simulink library "contactlib"  (R2013b)
settings: Solver=ode45  StartTime=0.0  StopTime=10.0  RelTol=1e-3
undefined symbols (not defined in the file): rWheel
libraries: nesl_utility x29, sm_lib x17, contactlib x4, dspinverses x2, contact3D_lib x2
settings Model: Creator=scastro  LastModifiedBy=scastro

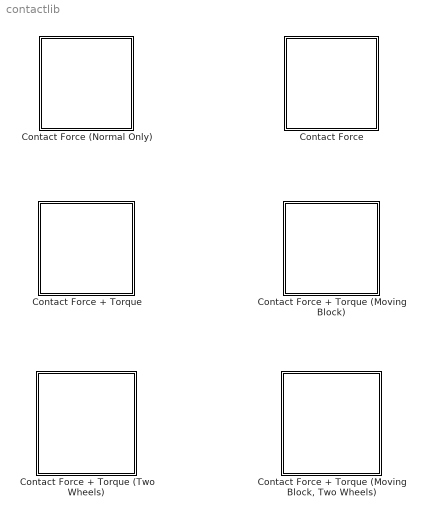
== system contactlib ==
  Contact Force : Subsystem  mask{rWheel=1, k=300000, b=5000, xBlock=2, yBlock=5, zBlock=0.2}
      mask prompts: rWheel "Wheel Radius [m]"; k "Contact Stiffness"; b "Contact Damping"; xBlock "Block X [m]"; yBlock "Block Y [m]"; zBlock "Block Z [m]"
  Contact Force (Normal Only) : Subsystem  mask{rWheel=1, k=500000, b=20000, xBlock=2, yBlock=3, zBlock=0.2}
      mask prompts: rWheel "Wheel Radius [m]"; k "Contact Stiffness"; b "Contact Damping"; xBlock "Block X [m]"; yBlock "Block Y [m]"; zBlock "Block Z [m]"
  Contact Force + Torque : Subsystem  mask{rWheel=rWheel, k=2500, b=100, b2=1000, xBlock=2, yBlock=3.5, zBlock=0.2}
      mask prompts: rWheel "Wheel Radius [m]"; k "Contact Stiffness"; b "Contact Damping"; b2 "Slip Damping"; xBlock "Block X [m]"; yBlock "Block Y [m]"; zBlock "Block Z [m]"
  Contact Force + Torque (Moving Block) : Subsystem  mask{rWheel=rWheel, k=2500, b=100, b2=0, xBlock=2, yBlock=3.5, zBlock=0.2}
      mask prompts: rWheel "Wheel Radius [m]"; k "Contact Stiffness"; b "Contact Damping"; b2 "Slip Damping"; xBlock "Block X [m]"; yBlock "Block Y [m]"; zBlock "Block Z [m]"
  "Contact Force + Torque (Moving Block, Two Wheels)" : Subsystem  AncestorBlock=|  mask{rWheel=0, k=0, b=0, b2=0, xBlock=0, yBlock=0, zBlock=0}
      | contactlib/Contact Force + Torque
      | (Two Wheels)
      mask prompts: rWheel "Wheel Radius [m]"; k "Contact Stiffness"; b "Contact Damping"; b2 "Slip Damping"; xBlock "Block X [m]"; yBlock "Block Y [m]"; zBlock "Block Z [m]"
  Contact Force + Torque (Two Wheels) : Subsystem  mask{rWheel=0, k=0, b=0, b2=0, xBlock=0, yBlock=0, zBlock=0}
      mask prompts: rWheel "Wheel Radius [m]"; k "Contact Stiffness"; b "Contact Damping"; b2 "Slip Damping"; xBlock "Block X [m]"; yBlock "Block Y [m]"; zBlock "Block Z [m]"

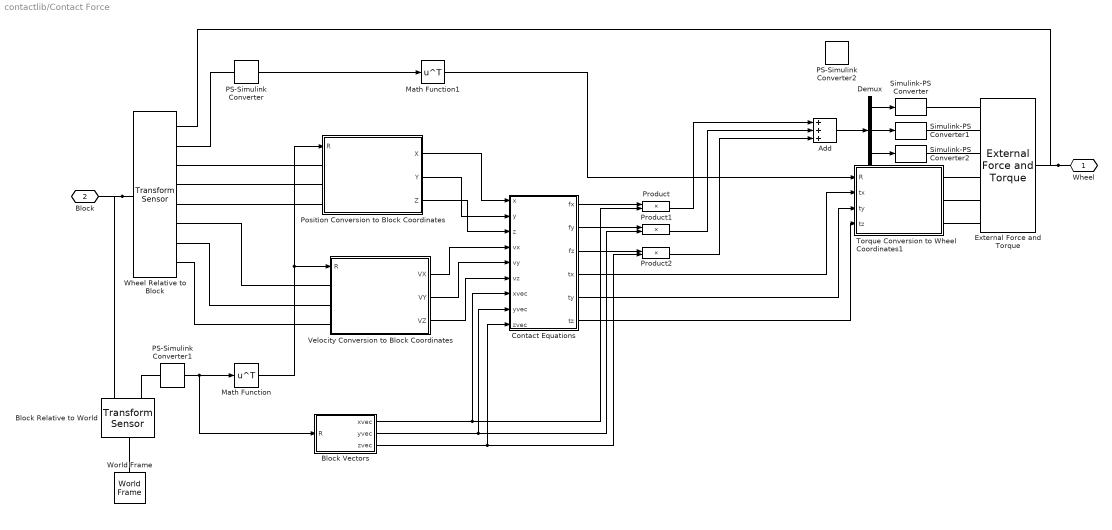
== system contactlib/Contact Force ==
  Add : Sum  Inputs=+++
  Block Relative to World : sm_lib/Frames and Transforms/Transform Sensor  MeasurementFrame=Base  SenseAngle=off  SenseAxis=off  SenseAngle1=off  SenseAngle2=off  SenseAngle3=off  SenseQ=off  SenseR=on  SenseOmegaX=off  SenseOmegaY=off  SenseOmegaZ=off  SenseOmega1=off  SenseOmega2=off  SenseOmega3=off  SenseQDot=off  SenseRDot=off  SenseAlphaX=off  SenseAlphaY=off  SenseAlphaZ=off  SenseAlpha1=off  SenseAlpha2=off  SenseAlpha3=off  SenseQDDot=off  SenseRDDot=off  SenseX=off  SenseY=off  SenseZ=off  SenseRad=off  SenseAzim=off  SenseDist=off  SenseInc=off  SenseXDot=off  SenseYDot=off  SenseZDot=off  SenseRadDot=off  SenseAzimDot=off  SenseDistDot=off  SenseIncDot=off  SenseXDDot=off  SenseYDDot=off  SenseZDDot=off  SenseRadDDot=off  SenseAzimDDot=off  SenseDistDDot=off  SenseIncDDot=off  BlockFunction=simmechanics.library.frames_transforms.transform_sensor
  Block Vectors : Subsystem
  Contact Equations : MATLAB Function  TreatAsAtomicUnit=on
  Demux : Demux  Outputs=3
  External Force and Torque : sm_lib/Forces and Torques/External Force and Torque  ForceResolutionFrame=World  EnableForceX=on  EnableForceY=on  EnableForceZ=on  EnableForce=off  TorqueResolutionFrame=AttachedFrame  EnableTorqueX=on  EnableTorqueY=on  EnableTorqueZ=on  EnableTorque=off  BlockFunction=simmechanics.library.forces_torques.external_force_torque
  Math Function : Math  Operator=transpose  SaturateOnIntegerOverflow=on
  Math Function1 : Math  Operator=transpose  SaturateOnIntegerOverflow=on
  PS-Simulink Converter : nesl_utility/PS-Simulink Converter  PhysicalDomain=network_engine_domain  SubClassName=ps_output  LeftPortType=input  RightPortType=output  PseudoPeriodic=off  Frequencies=[]  Unit=1  AffineConversion=off
  PS-Simulink Converter1 : nesl_utility/PS-Simulink Converter  PhysicalDomain=network_engine_domain  SubClassName=ps_output  LeftPortType=input  RightPortType=output  PseudoPeriodic=off  Frequencies=[]  Unit=1  AffineConversion=off
  PS-Simulink Converter2 : nesl_utility/PS-Simulink Converter  PhysicalDomain=network_engine_domain  SubClassName=ps_output  LeftPortType=input  RightPortType=output  PseudoPeriodic=off  Frequencies=[]  Unit=1  AffineConversion=off
  Position Conversion to Block Coordinates : Subsystem
  Product : Product
  Product1 : Product
  Product2 : Product
  Simulink-PS Converter : nesl_utility/Simulink-PS Converter  PhysicalDomain=network_engine_domain  SubClassName=ps_input  LeftPortType=input  RightPortType=output  PseudoPeriodic=off  Frequencies=[]  NoiseDistribution=none  NoiseParameters=[]  Unit=1  AffineConversion=off  InputFiltering=off  SimscapeFilterOrder=1  InputFilterTimeConstant=0.001  UdotUserProvided=1
  Simulink-PS Converter1 : nesl_utility/Simulink-PS Converter  PhysicalDomain=network_engine_domain  SubClassName=ps_input  LeftPortType=input  RightPortType=output  PseudoPeriodic=off  Frequencies=[]  NoiseDistribution=none  NoiseParameters=[]  Unit=1  AffineConversion=off  InputFiltering=off  SimscapeFilterOrder=1  InputFilterTimeConstant=0.001  UdotUserProvided=1
  Simulink-PS Converter2 : nesl_utility/Simulink-PS Converter  PhysicalDomain=network_engine_domain  SubClassName=ps_input  LeftPortType=input  RightPortType=output  PseudoPeriodic=off  Frequencies=[]  NoiseDistribution=none  NoiseParameters=[]  Unit=1  AffineConversion=off  InputFiltering=off  SimscapeFilterOrder=1  InputFilterTimeConstant=0.001  UdotUserProvided=1
  Torque Conversion to Wheel Coordinates1 : Subsystem
  Velocity Conversion to Block Coordinates : Subsystem
  Wheel Relative to Block : sm_lib/Frames and Transforms/Transform Sensor  MeasurementFrame=World  SenseAngle=off  SenseAxis=off  SenseAngle1=off  SenseAngle2=off  SenseAngle3=off  SenseQ=off  SenseR=on  SenseOmegaX=off  SenseOmegaY=off  SenseOmegaZ=off  SenseOmega1=off  SenseOmega2=off  SenseOmega3=off  SenseQDot=off  SenseRDot=off  SenseAlphaX=off  SenseAlphaY=off  SenseAlphaZ=off  SenseAlpha1=off  SenseAlpha2=off  SenseAlpha3=off  SenseQDDot=off  SenseRDDot=off  SenseX=on  SenseY=on  SenseZ=on  SenseRad=off  SenseAzim=off  SenseDist=off  SenseInc=off  SenseXDot=on  SenseYDot=on  SenseZDot=on  SenseRadDot=off  SenseAzimDot=off  SenseDistDot=off  SenseIncDot=off  SenseXDDot=off  SenseYDDot=off  SenseZDDot=off  SenseRadDDot=off  SenseAzimDDot=off  SenseDistDDot=off  SenseIncDDot=off  BlockFunction=simmechanics.library.frames_transforms.transform_sensor
  World Frame : sm_lib/Frames and Transforms/World Frame  BlockFunction=simmechanics.library.frames_transforms.world_frame
  Wheel : PMIOPort  Port=1  Side=Right
  Block : PMIOPort  Port=2  Side=Left
  wires:
  Math Function/1 -> Velocity Conversion to Block Coordinates/1(R), Position Conversion to Block Coordinates/1(R)
  PS-Simulink Converter1/1 -> Math Function/1, Block Vectors/1(R)
  Math Function1/1 -> Torque Conversion to Wheel Coordinates1/1(R)
  PS-Simulink Converter/1 -> Math Function1/1
  Contact Equations/3(fz) -> Product2/1
  Contact Equations/2(fy) -> Product1/1
  Contact Equations/1(fx) -> Product/1
  Velocity Conversion to Block Coordinates/3(VZ) -> Contact Equations/6(vz)
  Velocity Conversion to Block Coordinates/2(VY) -> Contact Equations/5(vy)
  Velocity Conversion to Block Coordinates/1(VX) -> Contact Equations/4(vx)
  Position Conversion to Block Coordinates/3(Z) -> Contact Equations/3(z)
  Position Conversion to Block Coordinates/2(Y) -> Contact Equations/2(y)
  Position Conversion to Block Coordinates/1(X) -> Contact Equations/1(x)
  Block Vectors/1(xvec) -> Contact Equations/7(xvec), Product/2
  Block Vectors/2(yvec) -> Contact Equations/8(yvec), Product1/2
  Block Vectors/3(zvec) -> Contact Equations/9(zvec), Product2/2
  Product/1 -> Add/1
  Product1/1 -> Add/2
  Product2/1 -> Add/3
  Add/1 -> Demux/1
  Demux/1 -> Simulink-PS Converter/1
  Demux/2 -> Simulink-PS Converter1/1
  Demux/3 -> Simulink-PS Converter2/1
  Contact Equations/4(tx) -> Torque Conversion to Wheel Coordinates1/2(tx)
  Contact Equations/5(ty) -> Torque Conversion to Wheel Coordinates1/3(ty)
  Contact Equations/6(tz) -> Torque Conversion to Wheel Coordinates1/4(tz)
  connections:
  Block Relative to World/RConn2 -- PS-Simulink Converter1/LConn1
  Wheel Relative to Block/RConn8 -- Velocity Conversion to Block Coordinates/LConn3
  Velocity Conversion to Block Coordinates/LConn2 -- Wheel Relative to Block/RConn7
  Wheel Relative to Block/RConn6 -- Velocity Conversion to Block Coordinates/LConn1
  Wheel Relative to Block/RConn5 -- Position Conversion to Block Coordinates/LConn3
  Position Conversion to Block Coordinates/LConn2 -- Wheel Relative to Block/RConn4
  Position Conversion to Block Coordinates/LConn1 -- Wheel Relative to Block/RConn3
  Wheel Relative to Block/RConn2 -- PS-Simulink Converter/LConn1
  Wheel Relative to Block/LConn1 -- Block Relative to World/RConn1 -- Block/RConn1
  Wheel/RConn1 -- Wheel Relative to Block/RConn1 -- External Force and Torque/RConn1
  Simulink-PS Converter/RConn1 -- External Force and Torque/LConn1
  Simulink-PS Converter1/RConn1 -- External Force and Torque/LConn2
  Simulink-PS Converter2/RConn1 -- External Force and Torque/LConn3
  Torque Conversion to Wheel Coordinates1/RConn1 -- External Force and Torque/LConn4
  External Force and Torque/LConn5 -- Torque Conversion to Wheel Coordinates1/RConn2
  Torque Conversion to Wheel Coordinates1/RConn3 -- External Force and Torque/LConn6
  World Frame/RConn1 -- Block Relative to World/LConn1

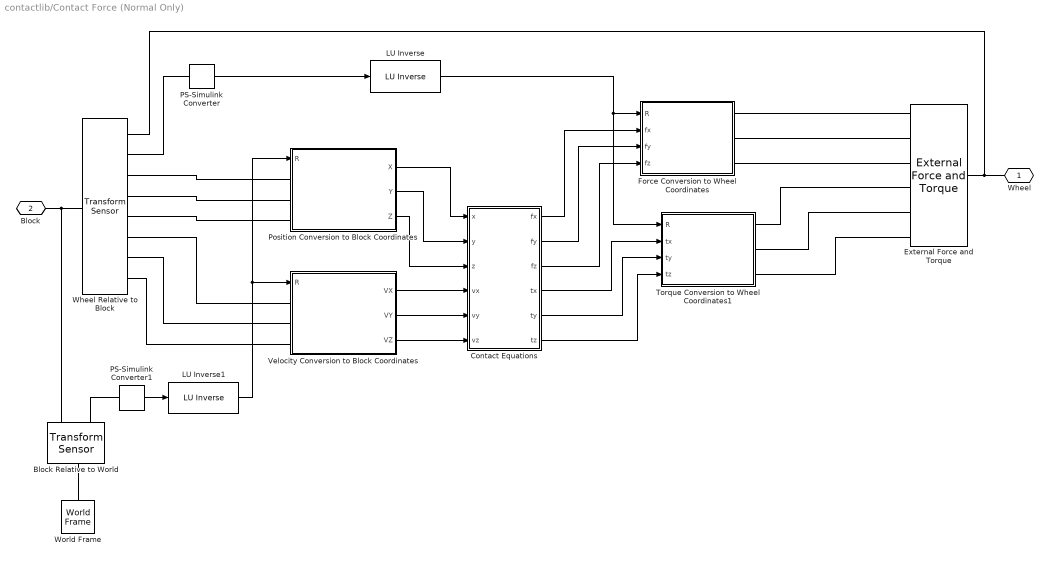
== system contactlib/Contact Force (Normal Only) ==
  " LU Inverse" : dspinverses/ LU Inverse
  " LU Inverse1" : dspinverses/ LU Inverse
  Block Relative to World : sm_lib/Frames and Transforms/Transform Sensor  MeasurementFrame=Base  SenseAngle=off  SenseAxis=off  SenseAngle1=off  SenseAngle2=off  SenseAngle3=off  SenseQ=off  SenseR=on  SenseOmegaX=off  SenseOmegaY=off  SenseOmegaZ=off  SenseOmega1=off  SenseOmega2=off  SenseOmega3=off  SenseQDot=off  SenseRDot=off  SenseAlphaX=off  SenseAlphaY=off  SenseAlphaZ=off  SenseAlpha1=off  SenseAlpha2=off  SenseAlpha3=off  SenseQDDot=off  SenseRDDot=off  SenseX=off  SenseY=off  SenseZ=off  SenseRad=off  SenseAzim=off  SenseDist=off  SenseInc=off  SenseXDot=off  SenseYDot=off  SenseZDot=off  SenseRadDot=off  SenseAzimDot=off  SenseDistDot=off  SenseIncDot=off  SenseXDDot=off  SenseYDDot=off  SenseZDDot=off  SenseRadDDot=off  SenseAzimDDot=off  SenseDistDDot=off  SenseIncDDot=off  BlockFunction=simmechanics.library.frames_transforms.transform_sensor
  Contact Equations : MATLAB Function  TreatAsAtomicUnit=on
  External Force and Torque : sm_lib/Forces and Torques/External Force and Torque  ForceResolutionFrame=AttachedFrame  EnableForceX=on  EnableForceY=on  EnableForceZ=on  EnableForce=off  TorqueResolutionFrame=AttachedFrame  EnableTorqueX=on  EnableTorqueY=on  EnableTorqueZ=on  EnableTorque=off  BlockFunction=simmechanics.library.forces_torques.external_force_torque
  Force Conversion to Wheel Coordinates : Subsystem
  PS-Simulink Converter : nesl_utility/PS-Simulink Converter  PhysicalDomain=network_engine_domain  SubClassName=ps_output  LeftPortType=input  RightPortType=output  PseudoPeriodic=off  Frequencies=[]  Unit=1  AffineConversion=off
  PS-Simulink Converter1 : nesl_utility/PS-Simulink Converter  PhysicalDomain=network_engine_domain  SubClassName=ps_output  LeftPortType=input  RightPortType=output  PseudoPeriodic=off  Frequencies=[]  Unit=1  AffineConversion=off
  Position Conversion to Block Coordinates : Subsystem
  Torque Conversion to Wheel Coordinates1 : Subsystem
  Velocity Conversion to Block Coordinates : Subsystem
  Wheel Relative to Block : sm_lib/Frames and Transforms/Transform Sensor  MeasurementFrame=World  SenseAngle=off  SenseAxis=off  SenseAngle1=off  SenseAngle2=off  SenseAngle3=off  SenseQ=off  SenseR=on  SenseOmegaX=off  SenseOmegaY=off  SenseOmegaZ=off  SenseOmega1=off  SenseOmega2=off  SenseOmega3=off  SenseQDot=off  SenseRDot=off  SenseAlphaX=off  SenseAlphaY=off  SenseAlphaZ=off  SenseAlpha1=off  SenseAlpha2=off  SenseAlpha3=off  SenseQDDot=off  SenseRDDot=off  SenseX=on  SenseY=on  SenseZ=on  SenseRad=off  SenseAzim=off  SenseDist=off  SenseInc=off  SenseXDot=on  SenseYDot=on  SenseZDot=on  SenseRadDot=off  SenseAzimDot=off  SenseDistDot=off  SenseIncDot=off  SenseXDDot=off  SenseYDDot=off  SenseZDDot=off  SenseRadDDot=off  SenseAzimDDot=off  SenseDistDDot=off  SenseIncDDot=off  BlockFunction=simmechanics.library.frames_transforms.transform_sensor
  World Frame : sm_lib/Frames and Transforms/World Frame  BlockFunction=simmechanics.library.frames_transforms.world_frame
  Wheel : PMIOPort  Port=1  Side=Right
  Block : PMIOPort  Port=2  Side=Left
  wires:
  Position Conversion to Block Coordinates/1(X) -> Contact Equations/1(x)
  Position Conversion to Block Coordinates/2(Y) -> Contact Equations/2(y)
  Position Conversion to Block Coordinates/3(Z) -> Contact Equations/3(z)
  Velocity Conversion to Block Coordinates/1(VX) -> Contact Equations/4(vx)
  Velocity Conversion to Block Coordinates/2(VY) -> Contact Equations/5(vy)
  Velocity Conversion to Block Coordinates/3(VZ) -> Contact Equations/6(vz)
  Contact Equations/1(fx) -> Force Conversion to Wheel Coordinates/2(fx)
  Contact Equations/2(fy) -> Force Conversion to Wheel Coordinates/3(fy)
  Contact Equations/3(fz) -> Force Conversion to Wheel Coordinates/4(fz)
  PS-Simulink Converter/1 -> " LU Inverse"/1
  " LU Inverse"/1 -> Torque Conversion to Wheel Coordinates1/1(R), Force Conversion to Wheel Coordinates/1(R)
  PS-Simulink Converter1/1 -> " LU Inverse1"/1
  Contact Equations/4(tx) -> Torque Conversion to Wheel Coordinates1/2(tx)
  Contact Equations/5(ty) -> Torque Conversion to Wheel Coordinates1/3(ty)
  Contact Equations/6(tz) -> Torque Conversion to Wheel Coordinates1/4(tz)
  " LU Inverse1"/1 -> Position Conversion to Block Coordinates/1(R), Velocity Conversion to Block Coordinates/1(R)
  connections:
  External Force and Torque/RConn1 -- Wheel Relative to Block/RConn1 -- Wheel/RConn1
  Block/RConn1 -- Block Relative to World/RConn1 -- Wheel Relative to Block/LConn1
  Wheel Relative to Block/RConn2 -- PS-Simulink Converter/LConn1
  Position Conversion to Block Coordinates/LConn1 -- Wheel Relative to Block/RConn3
  Position Conversion to Block Coordinates/LConn2 -- Wheel Relative to Block/RConn4
  Wheel Relative to Block/RConn5 -- Position Conversion to Block Coordinates/LConn3
  Wheel Relative to Block/RConn6 -- Velocity Conversion to Block Coordinates/LConn1
  Velocity Conversion to Block Coordinates/LConn2 -- Wheel Relative to Block/RConn7
  Wheel Relative to Block/RConn8 -- Velocity Conversion to Block Coordinates/LConn3
  Force Conversion to Wheel Coordinates/RConn1 -- External Force and Torque/LConn1
  Force Conversion to Wheel Coordinates/RConn2 -- External Force and Torque/LConn2
  External Force and Torque/LConn3 -- Force Conversion to Wheel Coordinates/RConn3
  World Frame/RConn1 -- Block Relative to World/LConn1
  Block Relative to World/RConn2 -- PS-Simulink Converter1/LConn1
  Torque Conversion to Wheel Coordinates1/RConn3 -- External Force and Torque/LConn6
  Torque Conversion to Wheel Coordinates1/RConn1 -- External Force and Torque/LConn4
  External Force and Torque/LConn5 -- Torque Conversion to Wheel Coordinates1/RConn2

== system contactlib/Contact Force + Torque ==
  Ball To Box 3D Contact : contact3D_lib/Ball To Box 3D Contact  rWheel=rWheel m  xBlock=xBlock m  yBlock=yBlock m  zBlock=zBlock m  k=k N/m  b=b N/(m/s)  b2=b2 N/(m/s)  F_Log=off  LocalVarNames=|F  LocalVarDescs=|F  LocalVarLogging=[]
  Block Relative to World : sm_lib/Frames and Transforms/Transform Sensor  MeasurementFrame=Base  SenseAngle=off  SenseAxis=off  SenseAngle1=off  SenseAngle2=off  SenseAngle3=off  SenseQ=off  SenseR=on  SenseOmegaX=off  SenseOmegaY=off  SenseOmegaZ=off  SenseOmega1=off  SenseOmega2=off  SenseOmega3=off  SenseQDot=off  SenseRDot=off  SenseAlphaX=off  SenseAlphaY=off  SenseAlphaZ=off  SenseAlpha1=off  SenseAlpha2=off  SenseAlpha3=off  SenseQDDot=off  SenseRDDot=off  SenseX=off  SenseY=off  SenseZ=off  SenseRad=off  SenseAzim=off  SenseDist=off  SenseInc=off  SenseXDot=off  SenseYDot=off  SenseZDot=off  SenseRadDot=off  SenseAzimDot=off  SenseDistDot=off  SenseIncDot=off  SenseXDDot=off  SenseYDDot=off  SenseZDDot=off  SenseRadDDot=off  SenseAzimDDot=off  SenseDistDDot=off  SenseIncDDot=off  BlockFunction=simmechanics.library.frames_transforms.transform_sensor
  External Force and Torque : sm_lib/Forces and Torques/External Force and Torque  ForceResolutionFrame=World  EnableForceX=off  EnableForceY=off  EnableForceZ=off  EnableForce=on  TorqueResolutionFrame=World  EnableTorqueX=off  EnableTorqueY=off  EnableTorqueZ=off  EnableTorque=on  BlockFunction=simmechanics.library.forces_torques.external_force_torque
  Wheel Relative to Block : sm_lib/Frames and Transforms/Transform Sensor  MeasurementFrame=Base  SenseAngle=off  SenseAxis=off  SenseAngle1=off  SenseAngle2=off  SenseAngle3=off  SenseQ=off  SenseR=on  SenseOmegaX=on  SenseOmegaY=on  SenseOmegaZ=on  SenseOmega1=off  SenseOmega2=off  SenseOmega3=off  SenseQDot=off  SenseRDot=off  SenseAlphaX=off  SenseAlphaY=off  SenseAlphaZ=off  SenseAlpha1=off  SenseAlpha2=off  SenseAlpha3=off  SenseQDDot=off  SenseRDDot=off  SenseX=on  SenseY=on  SenseZ=on  SenseRad=off  SenseAzim=off  SenseDist=off  SenseInc=off  SenseXDot=on  SenseYDot=on  SenseZDot=on  SenseRadDot=off  SenseAzimDot=off  SenseDistDot=off  SenseIncDot=off  SenseXDDot=off  SenseYDDot=off  SenseZDDot=off  SenseRadDDot=off  SenseAzimDDot=off  SenseDistDDot=off  SenseIncDDot=off  BlockFunction=simmechanics.library.frames_transforms.transform_sensor
  World Frame : sm_lib/Frames and Transforms/World Frame  BlockFunction=simmechanics.library.frames_transforms.world_frame
  Wheel : PMIOPort  Port=1  Side=Right
  Block : PMIOPort  Port=2  Side=Left
  connections:
  World Frame/RConn1 -- Block Relative to World/LConn1
  External Force and Torque/RConn1 -- Wheel/RConn1 -- Wheel Relative to Block/RConn1
  Block/RConn1 -- Block Relative to World/RConn1 -- Wheel Relative to Block/LConn1
  Ball To Box 3D Contact/RConn1 -- External Force and Torque/LConn1
  Ball To Box 3D Contact/RConn2 -- External Force and Torque/LConn2
  Block Relative to World/RConn2 -- Ball To Box 3D Contact/LConn1
  Ball To Box 3D Contact/LConn3 -- Wheel Relative to Block/RConn4
  Ball To Box 3D Contact/LConn4 -- Wheel Relative to Block/RConn5
  Ball To Box 3D Contact/LConn2 -- Wheel Relative to Block/RConn3
  Ball To Box 3D Contact/LConn7 -- Wheel Relative to Block/RConn8
  Ball To Box 3D Contact/LConn6 -- Wheel Relative to Block/RConn7
  Ball To Box 3D Contact/LConn5 -- Wheel Relative to Block/RConn6
  Wheel Relative to Block/RConn11 -- Ball To Box 3D Contact/LConn10
  Wheel Relative to Block/RConn10 -- Ball To Box 3D Contact/LConn9
  Wheel Relative to Block/RConn9 -- Ball To Box 3D Contact/LConn8

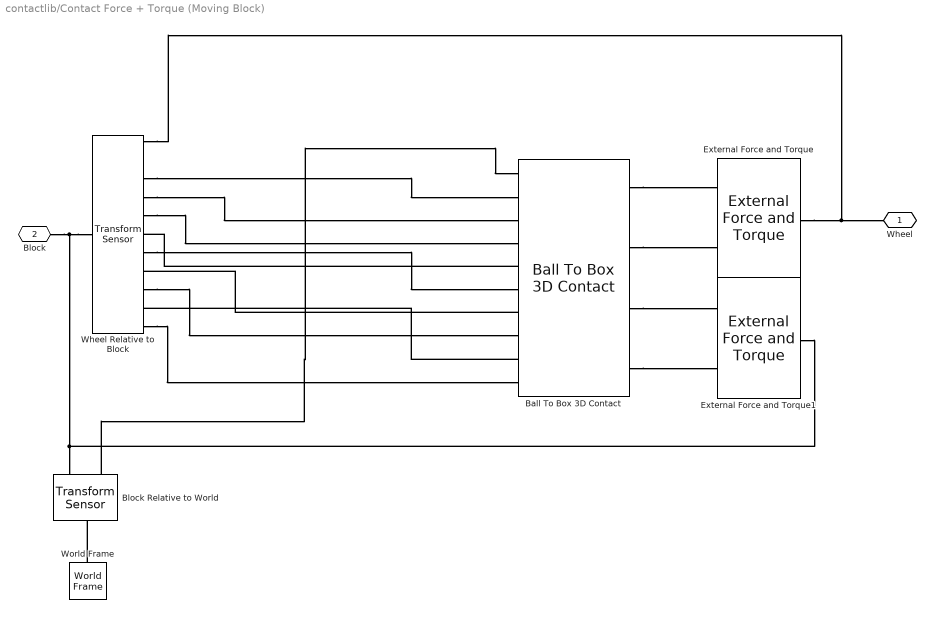
== system contactlib/Contact Force + Torque (Moving Block) ==
  Ball To Box 3D Contact : contact3D_lib/Ball To Box 3D Contact  rWheel=rWheel m  xBlock=xBlock m  yBlock=yBlock m  zBlock=zBlock m  k=k N/m  b=b N/(m/s)  b2=b2 N/(m/s)  F_Log=off  LocalVarNames=|F  LocalVarDescs=|F  LocalVarLogging=[]
  Block Relative to World : sm_lib/Frames and Transforms/Transform Sensor  MeasurementFrame=Base  SenseAngle=off  SenseAxis=off  SenseAngle1=off  SenseAngle2=off  SenseAngle3=off  SenseQ=off  SenseR=on  SenseOmegaX=off  SenseOmegaY=off  SenseOmegaZ=off  SenseOmega1=off  SenseOmega2=off  SenseOmega3=off  SenseQDot=off  SenseRDot=off  SenseAlphaX=off  SenseAlphaY=off  SenseAlphaZ=off  SenseAlpha1=off  SenseAlpha2=off  SenseAlpha3=off  SenseQDDot=off  SenseRDDot=off  SenseX=off  SenseY=off  SenseZ=off  SenseRad=off  SenseAzim=off  SenseDist=off  SenseInc=off  SenseXDot=off  SenseYDot=off  SenseZDot=off  SenseRadDot=off  SenseAzimDot=off  SenseDistDot=off  SenseIncDot=off  SenseXDDot=off  SenseYDDot=off  SenseZDDot=off  SenseRadDDot=off  SenseAzimDDot=off  SenseDistDDot=off  SenseIncDDot=off  BlockFunction=simmechanics.library.frames_transforms.transform_sensor
  External Force and Torque : sm_lib/Forces and Torques/External Force and Torque  ForceResolutionFrame=World  EnableForceX=off  EnableForceY=off  EnableForceZ=off  EnableForce=on  TorqueResolutionFrame=World  EnableTorqueX=off  EnableTorqueY=off  EnableTorqueZ=off  EnableTorque=on  BlockFunction=simmechanics.library.forces_torques.external_force_torque
  External Force and Torque1 : sm_lib/Forces and Torques/External Force and Torque  ForceResolutionFrame=AttachedFrame  EnableForceX=off  EnableForceY=off  EnableForceZ=off  EnableForce=on  TorqueResolutionFrame=AttachedFrame  EnableTorqueX=off  EnableTorqueY=off  EnableTorqueZ=off  EnableTorque=on  BlockFunction=simmechanics.library.forces_torques.external_force_torque
  Wheel Relative to Block : sm_lib/Frames and Transforms/Transform Sensor  MeasurementFrame=Base  SenseAngle=off  SenseAxis=off  SenseAngle1=off  SenseAngle2=off  SenseAngle3=off  SenseQ=off  SenseR=on  SenseOmegaX=on  SenseOmegaY=on  SenseOmegaZ=on  SenseOmega1=off  SenseOmega2=off  SenseOmega3=off  SenseQDot=off  SenseRDot=off  SenseAlphaX=off  SenseAlphaY=off  SenseAlphaZ=off  SenseAlpha1=off  SenseAlpha2=off  SenseAlpha3=off  SenseQDDot=off  SenseRDDot=off  SenseX=on  SenseY=on  SenseZ=on  SenseRad=off  SenseAzim=off  SenseDist=off  SenseInc=off  SenseXDot=on  SenseYDot=on  SenseZDot=on  SenseRadDot=off  SenseAzimDot=off  SenseDistDot=off  SenseIncDot=off  SenseXDDot=off  SenseYDDot=off  SenseZDDot=off  SenseRadDDot=off  SenseAzimDDot=off  SenseDistDDot=off  SenseIncDDot=off  BlockFunction=simmechanics.library.frames_transforms.transform_sensor
  World Frame : sm_lib/Frames and Transforms/World Frame  BlockFunction=simmechanics.library.frames_transforms.world_frame
  Wheel : PMIOPort  Port=1  Side=Right
  Block : PMIOPort  Port=2  Side=Left
  connections:
  Ball To Box 3D Contact/RConn4 -- External Force and Torque1/LConn2
  Ball To Box 3D Contact/RConn3 -- External Force and Torque1/LConn1
  Block Relative to World/RConn2 -- Ball To Box 3D Contact/LConn1
  Ball To Box 3D Contact/RConn2 -- External Force and Torque/LConn2
  Ball To Box 3D Contact/RConn1 -- External Force and Torque/LConn1
  Wheel Relative to Block/LConn1 -- External Force and Torque1/RConn1 -- Block Relative to World/RConn1 -- Block/RConn1
  Wheel Relative to Block/RConn1 -- Wheel/RConn1 -- External Force and Torque/RConn1
  World Frame/RConn1 -- Block Relative to World/LConn1
  Wheel Relative to Block/RConn3 -- Ball To Box 3D Contact/LConn2
  Wheel Relative to Block/RConn4 -- Ball To Box 3D Contact/LConn3
  Wheel Relative to Block/RConn5 -- Ball To Box 3D Contact/LConn4
  Ball To Box 3D Contact/LConn5 -- Wheel Relative to Block/RConn6
  Wheel Relative to Block/RConn7 -- Ball To Box 3D Contact/LConn6
  Ball To Box 3D Contact/LConn7 -- Wheel Relative to Block/RConn8
  Wheel Relative to Block/RConn9 -- Ball To Box 3D Contact/LConn8
  Ball To Box 3D Contact/LConn9 -- Wheel Relative to Block/RConn10
  Wheel Relative to Block/RConn11 -- Ball To Box 3D Contact/LConn10

== system contactlib/Contact Force + Torque (Moving Block, Two Wheels) ==
  Contact Force + Torque (Moving Block) : contactlib/Contact Force + Torque (Moving Block)  rWheel=rWheel  k=k  b=b  b2=b2  xBlock=xBlock  yBlock=yBlock  zBlock=zBlock
  Contact Force + Torque (Moving Block)1 : contactlib/Contact Force + Torque (Moving Block)  rWheel=rWheel  k=k  b=b  b2=b2  xBlock=xBlock  yBlock=yBlock  zBlock=zBlock
  L Wheel : PMIOPort  Port=1  Side=Right
  Block : PMIOPort  Port=2  Side=Left
  R Wheel : PMIOPort  Port=3  Side=Right
  connections:
  Contact Force + Torque (Moving Block)1/RConn1 -- R Wheel/RConn1
  Block/RConn1 -- Contact Force + Torque (Moving Block)1/LConn1 -- Contact Force + Torque (Moving Block)/LConn1
  Contact Force + Torque (Moving Block)/RConn1 -- L Wheel/RConn1

== system contactlib/Contact Force + Torque (Two Wheels) ==
  Contact Force + Torque : contactlib/Contact Force + Torque  rWheel=rWheel  k=k  b=b  b2=b2  xBlock=xBlock  yBlock=yBlock  zBlock=zBlock
  Contact Force + Torque1 : contactlib/Contact Force + Torque  rWheel=rWheel  k=k  b=b  b2=b2  xBlock=xBlock  yBlock=yBlock  zBlock=zBlock
  L Wheel : PMIOPort  Port=1  Side=Right
  Block : PMIOPort  Port=2  Side=Left
  R Wheel : PMIOPort  Port=3  Side=Right
  connections:
  Contact Force + Torque/RConn1 -- L Wheel/RConn1
  Contact Force + Torque/LConn1 -- Contact Force + Torque1/LConn1 -- Block/RConn1
  Contact Force + Torque1/RConn1 -- R Wheel/RConn1

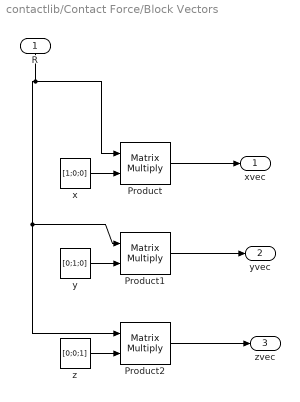
== system contactlib/Contact Force/Block Vectors ==
  R : Inport
  Product : Product  Multiplication=Matrix(*)
  Product1 : Product  Multiplication=Matrix(*)
  Product2 : Product  Multiplication=Matrix(*)
  x : Constant  Value=[1;0;0]
  y : Constant  Value=[0;1;0]
  z : Constant  Value=[0;0;1]
  xvec : Outport
  yvec : Outport  Port=2
  zvec : Outport  Port=3
  wires:
  Product1/1 -> yvec/1
  R/1 -> Product2/1, Product1/1, Product/1
  y/1 -> Product1/2
  x/1 -> Product/2
  Product/1 -> xvec/1
  Product2/1 -> zvec/1
  z/1 -> Product2/2

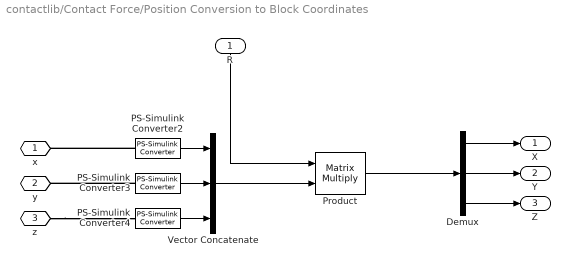
== system contactlib/Contact Force/Position Conversion to Block Coordinates ==
  R : Inport
  Demux : Demux  Outputs=3
  PS-Simulink Converter2 : nesl_utility/PS-Simulink Converter  PhysicalDomain=network_engine_domain  SubClassName=ps_output  LeftPortType=input  RightPortType=output  PseudoPeriodic=off  Frequencies=[]  Unit=1  AffineConversion=off
  PS-Simulink Converter3 : nesl_utility/PS-Simulink Converter  PhysicalDomain=network_engine_domain  SubClassName=ps_output  LeftPortType=input  RightPortType=output  PseudoPeriodic=off  Frequencies=[]  Unit=1  AffineConversion=off
  PS-Simulink Converter4 : nesl_utility/PS-Simulink Converter  PhysicalDomain=network_engine_domain  SubClassName=ps_output  LeftPortType=input  RightPortType=output  PseudoPeriodic=off  Frequencies=[]  Unit=1  AffineConversion=off
  Product : Product  Multiplication=Matrix(*)
  Vector Concatenate : Concatenate  NumInputs=3
  x : PMIOPort  Port=1  Side=Left
  y : PMIOPort  Port=2  Side=Left
  z : PMIOPort  Port=3  Side=Left
  X : Outport
  Y : Outport  Port=2
  Z : Outport  Port=3
  wires:
  Product/1 -> Demux/1
  R/1 -> Product/1
  PS-Simulink Converter2/1 -> Vector Concatenate/1
  PS-Simulink Converter3/1 -> Vector Concatenate/2
  Demux/1 -> X/1
  PS-Simulink Converter4/1 -> Vector Concatenate/3
  Demux/2 -> Y/1
  Demux/3 -> Z/1
  Vector Concatenate/1 -> Product/2
  connections:
  z/RConn1 -- PS-Simulink Converter4/LConn1
  PS-Simulink Converter3/LConn1 -- y/RConn1
  PS-Simulink Converter2/LConn1 -- x/RConn1

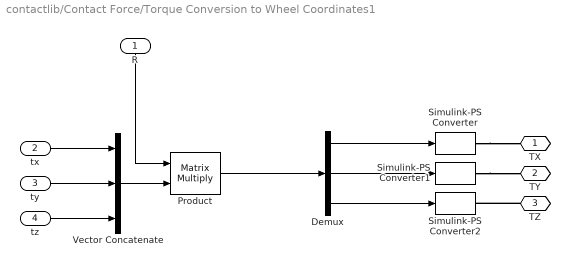
== system contactlib/Contact Force/Torque Conversion to Wheel Coordinates1 ==
  R : Inport
  tx : Inport  Port=2
  ty : Inport  Port=3
  tz : Inport  Port=4
  Demux : Demux  Outputs=3
  Product : Product  Multiplication=Matrix(*)
  Simulink-PS Converter : nesl_utility/Simulink-PS Converter  PhysicalDomain=network_engine_domain  SubClassName=ps_input  LeftPortType=input  RightPortType=output  PseudoPeriodic=off  Frequencies=[]  NoiseDistribution=none  NoiseParameters=[]  Unit=1  AffineConversion=off  InputFiltering=off  SimscapeFilterOrder=1  InputFilterTimeConstant=0.001  UdotUserProvided=1
  Simulink-PS Converter1 : nesl_utility/Simulink-PS Converter  PhysicalDomain=network_engine_domain  SubClassName=ps_input  LeftPortType=input  RightPortType=output  PseudoPeriodic=off  Frequencies=[]  NoiseDistribution=none  NoiseParameters=[]  Unit=1  AffineConversion=off  InputFiltering=off  SimscapeFilterOrder=1  InputFilterTimeConstant=0.001  UdotUserProvided=1
  Simulink-PS Converter2 : nesl_utility/Simulink-PS Converter  PhysicalDomain=network_engine_domain  SubClassName=ps_input  LeftPortType=input  RightPortType=output  PseudoPeriodic=off  Frequencies=[]  NoiseDistribution=none  NoiseParameters=[]  Unit=1  AffineConversion=off  InputFiltering=off  SimscapeFilterOrder=1  InputFilterTimeConstant=0.001  UdotUserProvided=1
  Vector Concatenate : Concatenate  NumInputs=3
  TX : PMIOPort  Port=1  Side=Right
  TY : PMIOPort  Port=2  Side=Right
  TZ : PMIOPort  Port=3  Side=Right
  wires:
  Vector Concatenate/1 -> Product/2
  tz/1 -> Vector Concatenate/3
  ty/1 -> Vector Concatenate/2
  tx/1 -> Vector Concatenate/1
  R/1 -> Product/1
  Demux/3 -> Simulink-PS Converter2/1
  Demux/2 -> Simulink-PS Converter1/1
  Demux/1 -> Simulink-PS Converter/1
  Product/1 -> Demux/1
  connections:
  Simulink-PS Converter/RConn1 -- TX/RConn1
  Simulink-PS Converter1/RConn1 -- TY/RConn1
  TZ/RConn1 -- Simulink-PS Converter2/RConn1

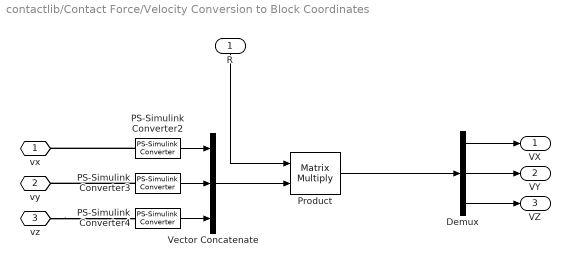
== system contactlib/Contact Force/Velocity Conversion to Block Coordinates ==
  R : Inport
  Demux : Demux  Outputs=3
  PS-Simulink Converter2 : nesl_utility/PS-Simulink Converter  PhysicalDomain=network_engine_domain  SubClassName=ps_output  LeftPortType=input  RightPortType=output  PseudoPeriodic=off  Frequencies=[]  Unit=1  AffineConversion=off
  PS-Simulink Converter3 : nesl_utility/PS-Simulink Converter  PhysicalDomain=network_engine_domain  SubClassName=ps_output  LeftPortType=input  RightPortType=output  PseudoPeriodic=off  Frequencies=[]  Unit=1  AffineConversion=off
  PS-Simulink Converter4 : nesl_utility/PS-Simulink Converter  PhysicalDomain=network_engine_domain  SubClassName=ps_output  LeftPortType=input  RightPortType=output  PseudoPeriodic=off  Frequencies=[]  Unit=1  AffineConversion=off
  Product : Product  Multiplication=Matrix(*)
  Vector Concatenate : Concatenate  NumInputs=3
  vx : PMIOPort  Port=1  Side=Left
  vy : PMIOPort  Port=2  Side=Left
  vz : PMIOPort  Port=3  Side=Left
  VX : Outport
  VY : Outport  Port=2
  VZ : Outport  Port=3
  wires:
  Product/1 -> Demux/1
  Vector Concatenate/1 -> Product/2
  Demux/3 -> VZ/1
  Demux/2 -> VY/1
  PS-Simulink Converter4/1 -> Vector Concatenate/3
  Demux/1 -> VX/1
  R/1 -> Product/1
  PS-Simulink Converter3/1 -> Vector Concatenate/2
  PS-Simulink Converter2/1 -> Vector Concatenate/1
  connections:
  PS-Simulink Converter2/LConn1 -- vx/RConn1
  PS-Simulink Converter3/LConn1 -- vy/RConn1
  vz/RConn1 -- PS-Simulink Converter4/LConn1

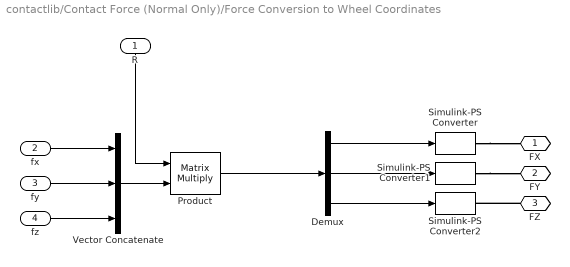
== system contactlib/Contact Force (Normal Only)/Force Conversion to Wheel Coordinates ==
  R : Inport
  fx : Inport  Port=2
  fy : Inport  Port=3
  fz : Inport  Port=4
  Demux : Demux  Outputs=3
  Product : Product  Multiplication=Matrix(*)
  Simulink-PS Converter : nesl_utility/Simulink-PS Converter  PhysicalDomain=network_engine_domain  SubClassName=ps_input  LeftPortType=input  RightPortType=output  PseudoPeriodic=off  Frequencies=[]  NoiseDistribution=none  NoiseParameters=[]  Unit=1  AffineConversion=off  InputFiltering=off  SimscapeFilterOrder=1  InputFilterTimeConstant=0.001  UdotUserProvided=1
  Simulink-PS Converter1 : nesl_utility/Simulink-PS Converter  PhysicalDomain=network_engine_domain  SubClassName=ps_input  LeftPortType=input  RightPortType=output  PseudoPeriodic=off  Frequencies=[]  NoiseDistribution=none  NoiseParameters=[]  Unit=1  AffineConversion=off  InputFiltering=off  SimscapeFilterOrder=1  InputFilterTimeConstant=0.001  UdotUserProvided=1
  Simulink-PS Converter2 : nesl_utility/Simulink-PS Converter  PhysicalDomain=network_engine_domain  SubClassName=ps_input  LeftPortType=input  RightPortType=output  PseudoPeriodic=off  Frequencies=[]  NoiseDistribution=none  NoiseParameters=[]  Unit=1  AffineConversion=off  InputFiltering=off  SimscapeFilterOrder=1  InputFilterTimeConstant=0.001  UdotUserProvided=1
  Vector Concatenate : Concatenate  NumInputs=3
  FX : PMIOPort  Port=1  Side=Right
  FY : PMIOPort  Port=2  Side=Right
  FZ : PMIOPort  Port=3  Side=Right
  wires:
  Vector Concatenate/1 -> Product/2
  fz/1 -> Vector Concatenate/3
  fy/1 -> Vector Concatenate/2
  fx/1 -> Vector Concatenate/1
  R/1 -> Product/1
  Demux/3 -> Simulink-PS Converter2/1
  Demux/2 -> Simulink-PS Converter1/1
  Demux/1 -> Simulink-PS Converter/1
  Product/1 -> Demux/1
  connections:
  Simulink-PS Converter/RConn1 -- FX/RConn1
  Simulink-PS Converter1/RConn1 -- FY/RConn1
  FZ/RConn1 -- Simulink-PS Converter2/RConn1

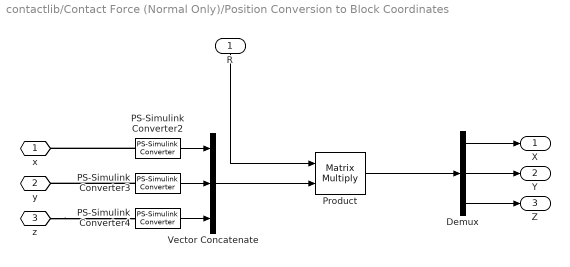
== system contactlib/Contact Force (Normal Only)/Position Conversion to Block Coordinates ==
  R : Inport
  Demux : Demux  Outputs=3
  PS-Simulink Converter2 : nesl_utility/PS-Simulink Converter  PhysicalDomain=network_engine_domain  SubClassName=ps_output  LeftPortType=input  RightPortType=output  PseudoPeriodic=off  Frequencies=[]  Unit=1  AffineConversion=off
  PS-Simulink Converter3 : nesl_utility/PS-Simulink Converter  PhysicalDomain=network_engine_domain  SubClassName=ps_output  LeftPortType=input  RightPortType=output  PseudoPeriodic=off  Frequencies=[]  Unit=1  AffineConversion=off
  PS-Simulink Converter4 : nesl_utility/PS-Simulink Converter  PhysicalDomain=network_engine_domain  SubClassName=ps_output  LeftPortType=input  RightPortType=output  PseudoPeriodic=off  Frequencies=[]  Unit=1  AffineConversion=off
  Product : Product  Multiplication=Matrix(*)
  Vector Concatenate : Concatenate  NumInputs=3
  x : PMIOPort  Port=1  Side=Left
  y : PMIOPort  Port=2  Side=Left
  z : PMIOPort  Port=3  Side=Left
  X : Outport
  Y : Outport  Port=2
  Z : Outport  Port=3
  wires:
  Vector Concatenate/1 -> Product/2
  Demux/3 -> Z/1
  Demux/2 -> Y/1
  PS-Simulink Converter4/1 -> Vector Concatenate/3
  Demux/1 -> X/1
  PS-Simulink Converter3/1 -> Vector Concatenate/2
  PS-Simulink Converter2/1 -> Vector Concatenate/1
  R/1 -> Product/1
  Product/1 -> Demux/1
  connections:
  PS-Simulink Converter2/LConn1 -- x/RConn1
  PS-Simulink Converter3/LConn1 -- y/RConn1
  z/RConn1 -- PS-Simulink Converter4/LConn1

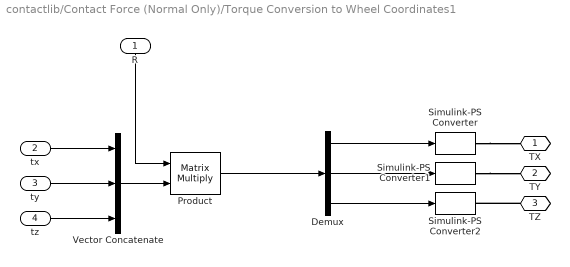
== system contactlib/Contact Force (Normal Only)/Torque Conversion to Wheel Coordinates1 ==
  R : Inport
  tx : Inport  Port=2
  ty : Inport  Port=3
  tz : Inport  Port=4
  Demux : Demux  Outputs=3
  Product : Product  Multiplication=Matrix(*)
  Simulink-PS Converter : nesl_utility/Simulink-PS Converter  PhysicalDomain=network_engine_domain  SubClassName=ps_input  LeftPortType=input  RightPortType=output  PseudoPeriodic=off  Frequencies=[]  NoiseDistribution=none  NoiseParameters=[]  Unit=1  AffineConversion=off  InputFiltering=off  SimscapeFilterOrder=1  InputFilterTimeConstant=0.001  UdotUserProvided=1
  Simulink-PS Converter1 : nesl_utility/Simulink-PS Converter  PhysicalDomain=network_engine_domain  SubClassName=ps_input  LeftPortType=input  RightPortType=output  PseudoPeriodic=off  Frequencies=[]  NoiseDistribution=none  NoiseParameters=[]  Unit=1  AffineConversion=off  InputFiltering=off  SimscapeFilterOrder=1  InputFilterTimeConstant=0.001  UdotUserProvided=1
  Simulink-PS Converter2 : nesl_utility/Simulink-PS Converter  PhysicalDomain=network_engine_domain  SubClassName=ps_input  LeftPortType=input  RightPortType=output  PseudoPeriodic=off  Frequencies=[]  NoiseDistribution=none  NoiseParameters=[]  Unit=1  AffineConversion=off  InputFiltering=off  SimscapeFilterOrder=1  InputFilterTimeConstant=0.001  UdotUserProvided=1
  Vector Concatenate : Concatenate  NumInputs=3
  TX : PMIOPort  Port=1  Side=Right
  TY : PMIOPort  Port=2  Side=Right
  TZ : PMIOPort  Port=3  Side=Right
  wires:
  Product/1 -> Demux/1
  Demux/1 -> Simulink-PS Converter/1
  Demux/2 -> Simulink-PS Converter1/1
  Demux/3 -> Simulink-PS Converter2/1
  R/1 -> Product/1
  tx/1 -> Vector Concatenate/1
  ty/1 -> Vector Concatenate/2
  tz/1 -> Vector Concatenate/3
  Vector Concatenate/1 -> Product/2
  connections:
  TZ/RConn1 -- Simulink-PS Converter2/RConn1
  Simulink-PS Converter1/RConn1 -- TY/RConn1
  Simulink-PS Converter/RConn1 -- TX/RConn1

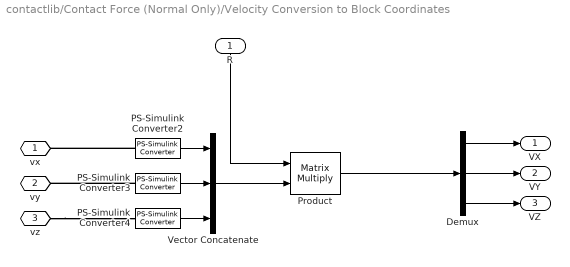
== system contactlib/Contact Force (Normal Only)/Velocity Conversion to Block Coordinates ==
  R : Inport
  Demux : Demux  Outputs=3
  PS-Simulink Converter2 : nesl_utility/PS-Simulink Converter  PhysicalDomain=network_engine_domain  SubClassName=ps_output  LeftPortType=input  RightPortType=output  PseudoPeriodic=off  Frequencies=[]  Unit=1  AffineConversion=off
  PS-Simulink Converter3 : nesl_utility/PS-Simulink Converter  PhysicalDomain=network_engine_domain  SubClassName=ps_output  LeftPortType=input  RightPortType=output  PseudoPeriodic=off  Frequencies=[]  Unit=1  AffineConversion=off
  PS-Simulink Converter4 : nesl_utility/PS-Simulink Converter  PhysicalDomain=network_engine_domain  SubClassName=ps_output  LeftPortType=input  RightPortType=output  PseudoPeriodic=off  Frequencies=[]  Unit=1  AffineConversion=off
  Product : Product  Multiplication=Matrix(*)
  Vector Concatenate : Concatenate  NumInputs=3
  vx : PMIOPort  Port=1  Side=Left
  vy : PMIOPort  Port=2  Side=Left
  vz : PMIOPort  Port=3  Side=Left
  VX : Outport
  VY : Outport  Port=2
  VZ : Outport  Port=3
  wires:
  PS-Simulink Converter2/1 -> Vector Concatenate/1
  PS-Simulink Converter3/1 -> Vector Concatenate/2
  R/1 -> Product/1
  Demux/1 -> VX/1
  PS-Simulink Converter4/1 -> Vector Concatenate/3
  Demux/2 -> VY/1
  Demux/3 -> VZ/1
  Vector Concatenate/1 -> Product/2
  Product/1 -> Demux/1
  connections:
  vz/RConn1 -- PS-Simulink Converter4/LConn1
  PS-Simulink Converter3/LConn1 -- vy/RConn1
  PS-Simulink Converter2/LConn1 -- vx/RConn1

== matlab function contactlib/Contact Force/Contact Equations ==
  data: x input; y input; z input; vx input; vy input; vz input; xvec input; yvec input; zvec input; fx output; fy output; fz output; tx output; ty output; tz output; rWheel parameter; xBlock parameter; yBlock parameter; zBlock parameter; k parameter; b parameter
function [fx, fy, fz, tx, ty, tz] = contact(x,y,z,vx,vy,vz,xvec,yvec,zvec, rWheel, xBlock, yBlock, zBlock, k, b)
%#codegen

fx = 0;
fy = 0;
fz = 0;
tx = 0;
ty = 0;
tz = 0;

% Logical Relationships
aboveLowerX = x > -(rWheel + xBlock/2);
belowUpperX = x < rWheel + xBlock/2;
insideX = (x<xBlock/2) && (x>-xBlock/2);

aboveLowerY = y > -(rWheel + yBlock/2);
belowUpperY = y < rWheel + yBlock/2;
insideY = (y<yBlock/2) && (y>-yBlock/2);

aboveLowerZ = z > -(rWheel + zBlock/2);
belowUpperZ = z < rWheel + zBlock/2;
insideZ = (z<zBlock/2) && (z>-zBlock/2);

% X direction
if insideY && insideZ && belowUpperX && aboveLowerX
        % Approaching from upper
        if abs(x-(rWheel+xBlock/2)) < abs(x+(rWheel+xBlock/2))
            fx = -k*(x - (rWheel+xBlock/2)) - b*vx;          
        % Approaching from lower
        else
            fx = -k*(rWheel+xBlock/2 + x) - b*vx;
        end
end

% Y direction
if insideX && insideZ && belowUpperY && aboveLowerY
        % Approaching from upper
        if abs(y-(rWheel+yBlock/2)) < abs(y+(rWheel+yBlock/2))
            fy = -k*(y - (rWheel+yBlock/2)) - b*vy;          
        % Approaching from lower
        else
            fy = -k*(rWheel+yBlock/2 + y) - b*vy;
        end
       
end

% Z direction
% NORMAL
if insideX && insideY && belowUpperZ && aboveLowerZ

        % Approaching from upper
        if abs(z-(rWheel+zBlock/2)) < abs(z+(rWheel+zBlock/2))
            fz = -k*(z - (rWheel+zBlock/2)) - b*vz;          
        % Approaching from lower
        else
            fz = -k*(rWheel+zBlock/2 + z) - b*vz;
        end
               
% UPPER RIGHT CORNER
elseif (insideX && ((y-yBlock/2)^2 + (z-zBlock/2)^2) < rWheel^2 )          

    theta = atan2(z-zBlock/2,y-yBlock/2);
    deltaZ = z - rWheel*sin(theta) - zBlock/2;
    fz = -k*deltaZ - b*vz;
    fy = fz/tan(theta);

% UPPER LEFT CORNER
elseif (insideX && ((y+yBlock/2)^2 + (z-zBlock/2)^2) < rWheel^2 )          

    theta = atan2(z-zBlock/2,y+yBlock/2);
    deltaZ = z - rWheel*sin(theta) - zBlock/2;
    fz = -k*deltaZ - b*vz;
    fy = fz/tan(theta);

end

end

== matlab function contactlib/Contact Force (Normal Only)/Contact Equations ==
  data: x input; y input; z input; vx input; vy input; vz input; fx output; fy output; fz output; tx output; ty output; tz output; rWheel parameter; xBlock parameter; yBlock parameter; zBlock parameter; k parameter; b parameter
function [fx, fy, fz, tx, ty, tz] = contact(x,y,z,vx,vy,vz, rWheel, xBlock, yBlock, zBlock, k, b)
%#codegen

fx = 0;
fy = 0;
fz = 0;
tx = 0;
ty = 0;
tz = 0;

% Logical Relationships
aboveLowerX = x > -(rWheel + xBlock/2);
belowUpperX = x < rWheel + xBlock/2;
insideX = (x<xBlock/2) && (x>-xBlock/2);

aboveLowerY = y > -(rWheel + yBlock/2);
belowUpperY = y < rWheel + yBlock/2;
insideY = (y<yBlock/2) && (y>-yBlock/2);

aboveLowerZ = z > -(rWheel + zBlock/2);
belowUpperZ = z < rWheel + zBlock/2;
insideZ = (z<zBlock/2) && (z>-zBlock/2);

% X direction
if insideY && insideZ && belowUpperX && aboveLowerX
        % Approaching from upper
        if abs(x-(rWheel+xBlock/2)) < abs(x+(rWheel+xBlock/2))
            fx = -k*(x - (rWheel+xBlock/2)) - b*vx;          
        % Approaching from lower
        else
            fx = -k*(rWheel+xBlock/2 + x) - b*vx;
        end
end

% Y direction
if insideX && insideZ && belowUpperY && aboveLowerY
        % Approaching from upper
        if abs(y-(rWheel+yBlock/2)) < abs(y+(rWheel+yBlock/2))
            fy = -k*(y - (rWheel+yBlock/2)) - b*vy;          
        % Approaching from lower
        else
            fy = -k*(rWheel+yBlock/2 + y) - b*vy;
        end
end

% Z direction
if insideX && insideY && belowUpperZ && aboveLowerZ
        % Approaching from upper
        if abs(z-(rWheel+zBlock/2)) < abs(z+(rWheel+zBlock/2))
            fz = -k*(z - (rWheel+zBlock/2)) - b*vz;          
        % Approaching from lower
        else
            fz = -k*(rWheel+zBlock/2 + z) - b*vz;
        end
end

end
